simulink model "Diagrama_de_Blocos_3"  (R2018b)
settings: Solver=FixedStepAuto  StartTime=0  StopTime=300  FixedStep=0.5e-3  RelTol=1e-3
undefined symbols (not defined in the file): A, hb, k1, k2, u1b, u2
settings Model: Creator=davi2  LastModifiedBy=davi2
settings DataIOCC: SaveFormat=Array  SaveOutput=off  SignalLogging=off  DSMLogging=off  TimeSaveName=t

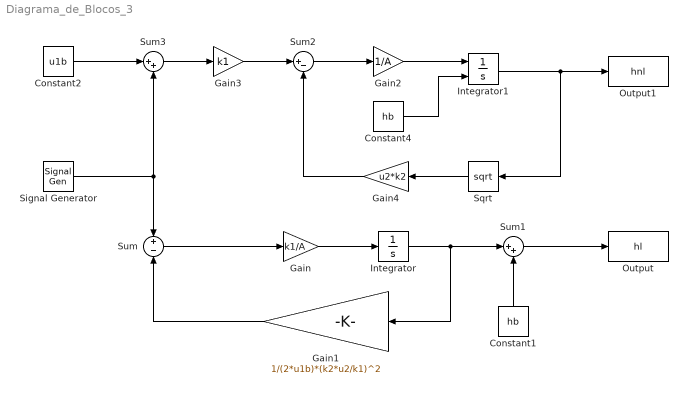
== system Diagrama_de_Blocos_3 ==
  Constant1 : Constant  Value=hb
  Constant2 : Constant  Value=u1b
  Constant4 : Constant  Value=hb
  Gain : Gain  Gain=k1/A
  Gain1 : Gain  Gain=1/(2*u1b)*(k2*u2/k1)^2
  Gain2 : Gain  Gain=1/A
  Gain3 : Gain  Gain=k1
  Gain4 : Gain  Gain=u2*k2
  Integrator : Integrator
  Integrator1 : Integrator  InitialConditionSource=external
  Output : ToWorkspace  VariableName=hl  SampleTime=-1
      settings: Save2DSignal=2-D array (concatenate along first dimension)
  Output1 : ToWorkspace  VariableName=hnl  SampleTime=-1
      settings: Save2DSignal=2-D array (concatenate along first dimension)
  Signal Generator : SignalGenerator  WaveForm=square  Amplitude=5
  Sqrt : Sqrt  SaturateOnIntegerOverflow=on
  Sum : Sum  Inputs=+|-
  Sum1 : Sum  Inputs=|++
  Sum2 : Sum  Inputs=|+-
  Sum3 : Sum  Inputs=|++
  wires:
  Sum1/1 -> Output/1
  Constant1/1 -> Sum1/2
  Constant4/1 -> Integrator1/2
  Constant2/1 -> Sum3/1
  Gain2/1 -> Integrator1/1
  Sqrt/1 -> Gain4/1
  Sum2/1 -> Gain2/1
  Sum3/1 -> Gain3/1
  Gain4/1 -> Sum2/2
  Integrator1/1 -> Output1/1, Sqrt/1
  Gain3/1 -> Sum2/1
  Signal Generator/1 -> Sum3/2, Sum/1
  Gain/1 -> Integrator/1
  Gain1/1 -> Sum/2
  Integrator/1 -> Sum1/1, Gain1/1
  Sum/1 -> Gain/1
